simulink model "gm_int2bin_sdi"  (R2024b)
settings: Solver=FixedStepDiscrete  StartTime=0.0  StopTime=9e3/100e6  RelTol=1e-3
libraries: hdlsllib x1
settings Model: PacingRate=0.001000  Creator=angro  LastModifiedBy=Angel
settings OptimizationCC: BlockReduction=off  ConditionallyExecuteInputs=off  DefaultParameterBehavior=Inlined  InheritOutputTypeSmallerThanSingle=on
settings DebuggingCC: AlgebraicLoopMsg=error  InheritedTsInSrcMsg=none  SingleTaskRateTransMsg=error  UnconnectedInputMsg=warning  UnconnectedOutputMsg=warning  UnconnectedLineMsg=warning  SFUnexpectedBacktrackingDiag=warning
settings HardwareCC: ProdBitPerPointer=32  ProdBitPerSizeT=32  ProdBitPerPtrDiffT=32  ProdLargestAtomicFloat=None  ProdIntDivRoundTo=Undefined  ProdEndianess=Unspecified  ProdWordSize=32  ProdHWDeviceType=ASIC/FPGA->ASIC/FPGA  TargetBitPerPointer=64  TargetBitPerSizeT=64  TargetBitPerPtrDiffT=64  TargetLongLongMode=on  TargetIntDivRoundTo=Zero  TargetEndianess=LittleEndian  TargetWordSize=64  TargetHWDeviceType=Custom Processor->MATLAB Host Computer  ProdEqTarget=off
settings RTWCC: GPUComputeCapability=3.5

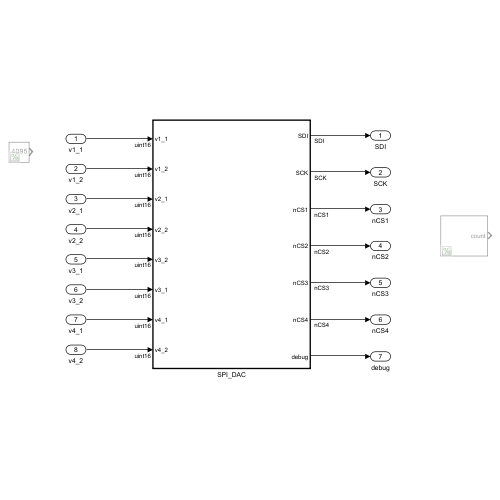
[thumbnail: Simulink's stored preview of the top-level diagram]
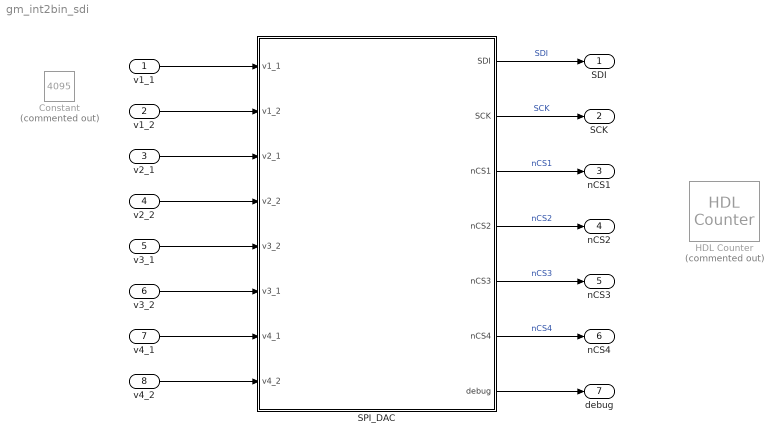
== system gm_int2bin_sdi ==
  v1_1 : Inport
  v1_2 : Inport  Port=2
  v2_1 : Inport  Port=3
  v2_2 : Inport  Port=4
  v3_1 : Inport  Port=5
  v3_2 : Inport  Port=6
  v4_1 : Inport  Port=7
  v4_2 : Inport  Port=8
  Constant : Constant  Commented=on  Value=4095  OutDataTypeStr=uint16
  HDL Counter : hdlsllib/Sources/HDL Counter  Commented=on  CountType=Count limited  CountInit=2040  CountStep=1  CountMax=2060  CountFromType=Initial value  CountFrom=2040  CountResetPort=off  CountLoadPort=off  CountEnbPort=off  CountDirPort=off  CountHitOutputPort=off  CountDataType=Unsigned  CountWordLen=16  CountFracLen=0  CountSampTime=-1
  SPI_DAC : Subsystem  TreatAsAtomicUnit=on
  SDI : Outport
  SCK : Outport  Port=2
  nCS1 : Outport  Port=3
  nCS2 : Outport  Port=4
  nCS3 : Outport  Port=5
  nCS4 : Outport  Port=6
  debug : Outport  Port=7
  wires:
  v1_1/1 -> SPI_DAC/1(v1_1)
  SPI_DAC/7(debug) -> debug/1
  SPI_DAC/6(nCS4) -> nCS4/1  "nCS4"
  SPI_DAC/2(SCK) -> SCK/1  "SCK"
  SPI_DAC/3(nCS1) -> nCS1/1  "nCS1"
  SPI_DAC/1(SDI) -> SDI/1  "SDI"
  v4_2/1 -> SPI_DAC/8(v4_2)
  v4_1/1 -> SPI_DAC/7(v4_1)
  v3_1/1 -> SPI_DAC/5(v3_2)
  v2_2/1 -> SPI_DAC/4(v2_2)
  SPI_DAC/4(nCS2) -> nCS2/1  "nCS2"
  SPI_DAC/5(nCS3) -> nCS3/1  "nCS3"
  v2_1/1 -> SPI_DAC/3(v2_1)
  v1_2/1 -> SPI_DAC/2(v1_2)
  v3_2/1 -> SPI_DAC/6(v3_1)

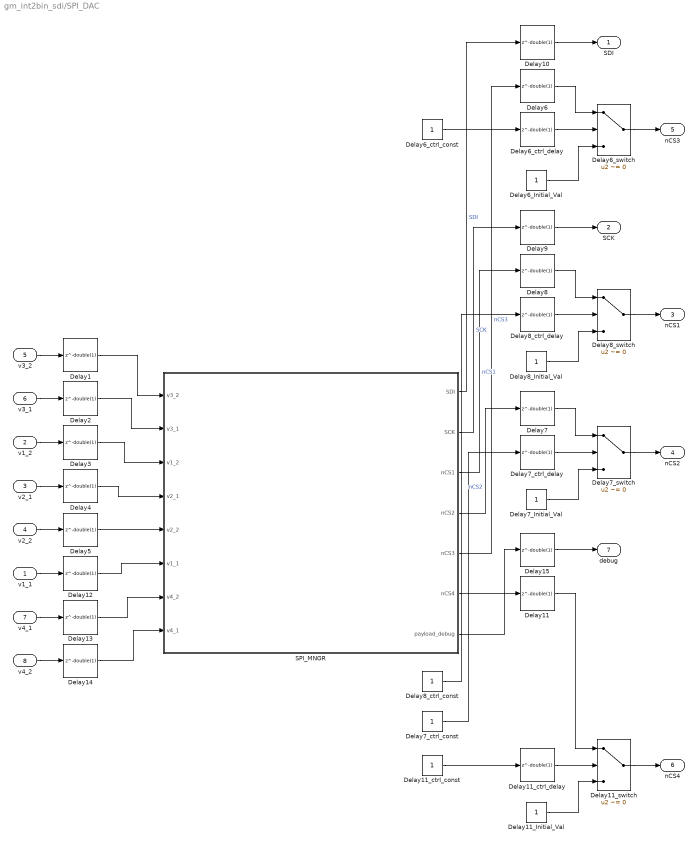
== system gm_int2bin_sdi/SPI_DAC ==
  v1_1 : Inport  OutDataTypeStr=uint16  PortDimensions=1  SampleTime=1.8e-06
  v1_2 : Inport  Port=2  OutDataTypeStr=uint16  PortDimensions=1  SampleTime=1.8e-06
  v2_1 : Inport  Port=3  OutDataTypeStr=uint16  PortDimensions=1  SampleTime=1.8e-06
  v2_2 : Inport  Port=4  OutDataTypeStr=uint16  PortDimensions=1  SampleTime=1.8e-06
  v3_2 : Inport  Port=5  OutDataTypeStr=uint16  PortDimensions=1  SampleTime=1.8e-06
  v3_1 : Inport  Port=6  OutDataTypeStr=uint16  PortDimensions=1  SampleTime=1.8e-06
  v4_1 : Inport  Port=7  OutDataTypeStr=uint16  PortDimensions=1  SampleTime=1.8e-06
  v4_2 : Inport  Port=8  OutDataTypeStr=uint16  PortDimensions=1  SampleTime=1.8e-06
  Delay{1..15} (15 alike) : Delay  DelayLength=double(1)  InitialCondition=0  SampleTime=1.8e-06
  Delay11_Initial_Val : Constant  OutDataTypeStr=boolean  SampleTime=1.8e-06
  Delay11_ctrl_const : Constant  OutDataTypeStr=boolean  SampleTime=1.8e-06
  Delay11_ctrl_delay : Delay  DelayLength=double(1)  InitialCondition=0  SampleTime=1.8e-06
  Delay11_switch : Switch  Criteria=u2 ~= 0  Threshold=double(0)  OutDataTypeStr=boolean  SampleTime=1.8e-06  SaturateOnIntegerOverflow=off  InputSameDT=off
  Delay6_Initial_Val : Constant  OutDataTypeStr=boolean  SampleTime=1.8e-06
  Delay6_ctrl_const : Constant  OutDataTypeStr=boolean  SampleTime=1.8e-06
  Delay6_ctrl_delay : Delay  DelayLength=double(1)  InitialCondition=0  SampleTime=1.8e-06
  Delay6_switch : Switch  Criteria=u2 ~= 0  Threshold=double(0)  OutDataTypeStr=boolean  SampleTime=1.8e-06  SaturateOnIntegerOverflow=off  InputSameDT=off
  Delay7_Initial_Val : Constant  OutDataTypeStr=boolean  SampleTime=1.8e-06
  Delay7_ctrl_const : Constant  OutDataTypeStr=boolean  SampleTime=1.8e-06
  Delay7_ctrl_delay : Delay  DelayLength=double(1)  InitialCondition=0  SampleTime=1.8e-06
  Delay7_switch : Switch  Criteria=u2 ~= 0  Threshold=double(0)  OutDataTypeStr=boolean  SampleTime=1.8e-06  SaturateOnIntegerOverflow=off  InputSameDT=off
  Delay8_Initial_Val : Constant  OutDataTypeStr=boolean  SampleTime=1.8e-06
  Delay8_ctrl_const : Constant  OutDataTypeStr=boolean  SampleTime=1.8e-06
  Delay8_ctrl_delay : Delay  DelayLength=double(1)  InitialCondition=0  SampleTime=1.8e-06
  Delay8_switch : Switch  Criteria=u2 ~= 0  Threshold=double(0)  OutDataTypeStr=boolean  SampleTime=1.8e-06  SaturateOnIntegerOverflow=off  InputSameDT=off
  SPI_MNGR : Stateflow chart  TreatAsAtomicUnit=on
  SDI : Outport  SampleTime=1.8e-06
  SCK : Outport  Port=2  SampleTime=1.8e-06
  nCS1 : Outport  Port=3  SampleTime=1.8e-06
  nCS2 : Outport  Port=4  SampleTime=1.8e-06
  nCS3 : Outport  Port=5  SampleTime=1.8e-06
  nCS4 : Outport  Port=6  SampleTime=1.8e-06
  debug : Outport  Port=7  SampleTime=1.8e-06
  wires:
  v2_1/1 -> Delay4/1
  v4_1/1 -> Delay13/1
  v2_2/1 -> Delay5/1
  v3_1/1 -> Delay2/1
  v1_2/1 -> Delay3/1
  v3_2/1 -> Delay1/1
  v1_1/1 -> Delay12/1
  v4_2/1 -> Delay14/1
  Delay13/1 -> SPI_MNGR/7(v4_2)
  Delay1/1 -> SPI_MNGR/1(v3_2)
  Delay2/1 -> SPI_MNGR/2(v3_1)
  Delay3/1 -> SPI_MNGR/3(v1_2)
  Delay4/1 -> SPI_MNGR/4(v2_1)
  Delay15/1 -> debug/1
  Delay5/1 -> SPI_MNGR/5(v2_2)
  Delay12/1 -> SPI_MNGR/6(v1_1)
  Delay10/1 -> SDI/1
  Delay14/1 -> SPI_MNGR/8(v4_1)
  Delay11_switch/1 -> nCS4/1
  Delay6_ctrl_const/1 -> Delay6_ctrl_delay/1
  SPI_MNGR/5(nCS3) -> Delay6/1  "nCS3"
  SPI_MNGR/1(SDI) -> Delay10/1  "SDI"
  SPI_MNGR/6(nCS4) -> Delay11/1
  SPI_MNGR/2(SCK) -> Delay9/1  "SCK"
  SPI_MNGR/3(nCS1) -> Delay8/1  "nCS1"
  SPI_MNGR/4(nCS2) -> Delay7/1  "nCS2"
  SPI_MNGR/7(payload_debug) -> Delay15/1
  Delay8_switch/1 -> nCS1/1
  Delay8_ctrl_const/1 -> Delay8_ctrl_delay/1
  Delay7_switch/1 -> nCS2/1
  Delay6_switch/1 -> nCS3/1
  Delay7_ctrl_const/1 -> Delay7_ctrl_delay/1
  Delay9/1 -> SCK/1
  Delay11_ctrl_const/1 -> Delay11_ctrl_delay/1
  Delay6/1 -> Delay6_switch/1
  Delay11_ctrl_delay/1 -> Delay11_switch/2
  Delay6_ctrl_delay/1 -> Delay6_switch/2
  Delay6_Initial_Val/1 -> Delay6_switch/3
  Delay8/1 -> Delay8_switch/1
  Delay8_ctrl_delay/1 -> Delay8_switch/2
  Delay8_Initial_Val/1 -> Delay8_switch/3
  Delay11_Initial_Val/1 -> Delay11_switch/3
  Delay7/1 -> Delay7_switch/1
  Delay7_ctrl_delay/1 -> Delay7_switch/2
  Delay7_Initial_Val/1 -> Delay7_switch/3
  Delay11/1 -> Delay11_switch/1

== stateflow chart gm_int2bin_sdi/SPI_DAC/SPI_MNGR ==
  settings: executeAtInitialization=1
  state on
    SDI=false;
    SCK=false;
    nCS1=true;
    nCS2=true;
    nCS3=true;
    nCS4=true;
    selector = 1;
  state off
    r_v11 = v1_1;
    r_v12 = v1_2;
    r_v21 = v2_1;
    r_v22 = v2_2;
    r_v31 = v3_1;
    r_v32 = v3_2;
    r_v41 = v4_1;
    r_v42 = v4_2;
  state toBsend_v1_1
    cont_bits = [simfcn1(r_v11)]';
    payload=[false true true true cont_bits(1:12)']';
    nCS1=false;
    nCS2=true;
    nCS3=true;
    nCS4=true;
  state toBsend_v1_2
    cont_bits_12 = [simfcn1(r_v12)]';
    payload=[true true true true cont_bits_12(1:12)']';
    nCS1=false;
    nCS2=true;
    nCS3=true;
    nCS4=true;
  state toBsend_v2_1
    cont_bits_21 = [simfcn1(r_v21)]';
    payload=[false true true true cont_bits_21(1:12)']';
    nCS1=true;
    nCS2=false;
    nCS3=true;
    nCS4=true;
  state toBsend_v2_2
    cont_bits_22 = [simfcn1(r_v22)]';
    payload=[true true true true cont_bits_22(1:12)']';
    nCS1=true;
    nCS2=false;
    nCS3=true;
    nCS4=true;
  state toBsend_v3_1
    cont_bits_31 = [simfcn1(r_v31)]';
    payload=[false true true true cont_bits_31(1:12)']';
    nCS1=true;
    nCS2=true;
    nCS3=false;
    nCS4=true;
  state toBsend_v3_2
    cont_bits_32 = [simfcn1(r_v32)]';
    payload=[true true true true cont_bits_32(1:12)']';
    nCS1=true;
    nCS2=true;
    nCS3=false;
    nCS4=true;
  state toBsend_v4_1
    cont_bits_41 = [simfcn1(r_v41)]';
    payload=[false true true true cont_bits_41(1:12)']';
    nCS1=true;
    nCS2=true;
    nCS3=true;
    nCS4=false;
  state toBsend_v3_3
    cont_bits_42 = [simfcn1(r_v42)]';
    payload=[true true true true cont_bits_42(1:12)']';
    nCS1=true;
    nCS2=true;
    nCS3=true;
    nCS4=false;
  state sender_pre_SCK
    SDI=payload(cnt);
    SCK=false;
  state sender_at_SCK
    SDI=payload(cnt);
    SCK=true;
  state NOP
    SCK=false;
  state sender_at_SCK1
    SDI=false;
    nCS1=true;
    nCS2=true;
    nCS3=true;
    nCS4=true;
    payload_debug= payload;
  state NOP1
  (default) -> on
  (junction 431) -> on [order 2] : [selector==8]
  on -> off
  (junction 431) -> (junction 300) [order 1] : [selector<8]{selector=selector+1;}
  (junction 429) -> (junction 431)
  off -> (junction 300)
  (junction 300) -> (junction 520) [order 2]
  (junction 520) -> (junction 632) [order 2]
  (junction 632) -> (junction 634) [order 2]
  (junction 634) -> (junction 636) [order 2]
  (junction 636) -> (junction 638) [order 2]
  (junction 638) -> (junction 649) [order 2]
  (junction 649) -> (junction 650) [order 1]
  (junction 300) -> (junction 645) [order 3]
  (junction 300) -> toBsend_v1_1 [order 1] : [selector==1]
  (junction 520) -> toBsend_v1_2 [order 1] : [selector==2]
  (junction 632) -> toBsend_v2_1 [order 1] : [selector==3]
  (junction 634) -> toBsend_v2_2 [order 1] : [selector==4]
  (junction 636) -> toBsend_v3_1 [order 1] : [selector==5]
  (junction 638) -> toBsend_v3_2 [order 1] : [selector==6]
  (junction 649) -> toBsend_v4_1 [order 2] : [selector==7
      | ]
  (junction 650) -> toBsend_v3_3 : [selector==8
      | ]
  toBsend_v1_1 -> (junction 516)
  toBsend_v1_2 -> (junction 535)
  toBsend_v2_1 -> (junction 703)
  toBsend_v2_2 -> (junction 716)
  toBsend_v3_1 -> (junction 722)
  toBsend_v3_2 -> (junction 725)
  toBsend_v4_1 -> (junction 732)
  toBsend_v3_3 -> (junction 734)
  (junction 535) -> (junction 516)
  (junction 703) -> (junction 535)
  (junction 716) -> (junction 703)
  (junction 722) -> (junction 716)
  (junction 725) -> (junction 722)
  (junction 732) -> (junction 725)
  (junction 734) -> (junction 732)
  (junction 516) -> sender_pre_SCK
  (junction 424) -> sender_pre_SCK : {cnt=cnt+1;}
  (junction 422) -> (junction 424)
  sender_pre_SCK -> (junction 405)
  (junction 407) -> sender_pre_SCK
  (junction 405) -> (junction 407) [order 1] : [cnt_clk<=2]{cnt_clk=cnt_clk+1;}
  (junction 405) -> sender_at_SCK [order 2] : [cnt_clk>2]{cnt_clk=1;}
  sender_at_SCK -> (junction 416)
  (junction 418) -> sender_at_SCK
  (junction 416) -> (junction 418) [order 2] : [cnt_clk<=2]{cnt_clk=cnt_clk+1;}
  (junction 416) -> (junction 421) [order 1] : [cnt_clk>2]{cnt_clk=1;}
  (junction 421) -> (junction 422) [order 2]
  (junction 421) -> NOP [order 1] : [cnt>=16]{cnt=1;}
  NOP -> (junction 613)
  (junction 616) -> NOP
  (junction 613) -> (junction 616) [order 2] : [cnt_clk<=2]{cnt_clk=cnt_clk+1;}
  (junction 613) -> sender_at_SCK1 [order 1] : [cnt_clk>2]{cnt_clk=1;}
  sender_at_SCK1 -> (junction 611)
  (junction 609) -> sender_at_SCK1
  (junction 611) -> (junction 609) [order 1] : [cnt_clk<=2]{cnt_clk=cnt_clk+1;}
  (junction 611) -> (junction 427) [order 2] : [cnt_clk>2]{cnt_clk=1;}
  (junction 623) -> (junction 429)
  (junction 427) -> NOP1 : {SCK=false;}
  NOP1 -> (junction 620)
  (junction 624) -> NOP1
  (junction 620) -> (junction 623) [order 2] : [cnt_clk>6]{cnt_clk=1;}
  (junction 620) -> (junction 624) [order 1] : [cnt_clk<=6]{cnt_clk=cnt_clk+1;}
  data: vx function_input; cont_bits2 function_output; v3_2 input; v3_1 input; v1_2 input; v2_1 input; v2_2 input; SDI output boolean; SCK output boolean; nCS1 output boolean =true; nCS2 output boolean =true; nCS3 output boolean =true; v1_1 input uint16 size=1; cnt local uint16 =1; cnt_clk local uint16 =1; payload local boolean size=16; selector local uint16 =1; cont_bits local boolean size=12; nCS4 output; v4_2 input; v4_1 input; r_v11 local; r_v42 local; r_v32 local; r_v41 local; r_v12 local; r_v21 local; r_v22 local; r_v31 local; payload_debug output; cont_bits_12 local; cont_bits_21 local; cont_bits_22 local; cont_bits_31 local; cont_bits_32 local; cont_bits_41 local; cont_bits_42 local
  function cont_bits2 = simfcn1(vx):
    | function cont_bits2 = simfcn1(vx)
    | 
    |     % cont_bits2 = int2bit(vx,12,1);
    | cont_bits2  = zeros(1,12)&0;
    | all_1 = uint16(0b1);
    | cont_bits2(12) = bitshift(bitand(all_1,vx),0);
    | 
    | all_2 = uint16(0b10);
    | cont_bits2(11) =bitshift(bitand(all_2,vx),-1);
    | 
    | all_3 = uint16(0b100);
    | cont_bits2(10) =bitshift(bitand(all_3,vx),-2);
    | 
    | all_4 = uint16(0b1000);
    | cont_bits2(9) =bitshift(bitand(all_4,vx),-3);
    | 
    | all_5 = uint16(0b10000);
    | cont_bits2(8) =bitshift(bitand(all_5,vx),-4);
    | 
    | all_6 = uint16(0b100000);
    | cont_bits2(7) =bitshift(bitand(all_6,vx),-5);
    | 
    | all_7 = uint16(0b1000000);
    | cont_bits2(6) =bitshift(bitand(all_7,vx),-6);
    | 
    | all_8 = uint16(0b10000000);
    | cont_bits2(5) =bitshift(bitand(all_8,vx),-7);
    | 
    | all_9 = uint16(0b100000000);
    | cont_bits2(4) =bitshift(bitand(all_9,vx),-8);
    | 
    | all_10 = uint16(0b1000000000);
    | cont_bits2(3) =bitshift(bitand(all_10,vx),-9);
    | 
    | all_11 = uint16(0b10000000000);
    | cont_bits2(2) =bitshift(bitand(all_11,vx),-10);
    | 
    | all_12 = uint16(0b100000000000);
    | cont_bits2(1) =bitshift(bitand(all_12,vx),-11);
    |   
    | 
    | end
